simulink subsystem "Car"  (R2022b)
settings: Solver=VariableStepAuto  StartTime=0.0  StopTime=10.0  RelTol=1e-3
model mask{InitPos=0, InitVol=0}
  mask prompts: InitPos "Initial position (m)"; InitVol "Initial velocity (Km/hr)"
undefined symbols (not defined in the file or in its folder): DiscIntNeverNeededParam
settings Model: Creator=MAAM  LastModifiedBy=MAAM

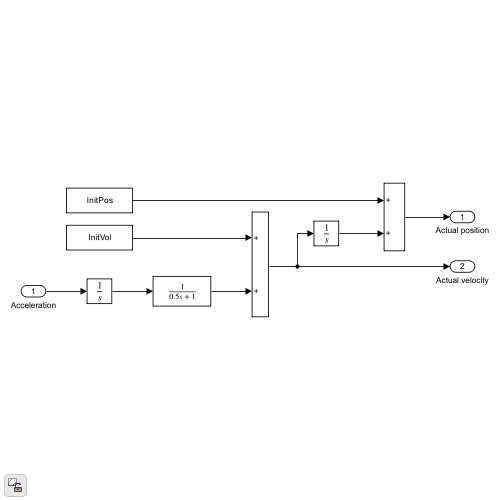
[thumbnail: Simulink's stored preview of the top-level diagram]
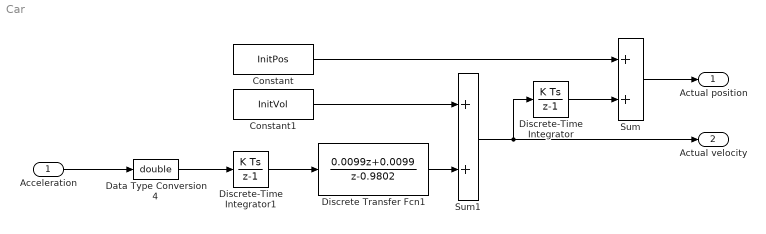
== system Car ==
  Acceleration : Inport
  Constant : Constant  Value=InitPos  OutDataTypeStr=Inherit: Inherit via back propagation  SampleTime=-1
  Constant1 : Constant  Value=InitVol  OutDataTypeStr=Inherit: Inherit via back propagation  SampleTime=-1
  Data Type Conversion4 : DataTypeConversion  OutDataTypeStr=double  SaturateOnIntegerOverflow=off  RndMeth=Floor
  Discrete Transfer Fcn1 : DiscreteTransferFcn  Numerator=[0.0099 0.0099]  Denominator=[1 -0.9802]  SampleTime=0.01
  Discrete-Time Integrator : DiscreteIntegrator  SampleTime=-1  ICPrevOutput=DiscIntNeverNeededParam  ICPrevScaledInput=DiscIntNeverNeededParam
  Discrete-Time Integrator1 : DiscreteIntegrator  SampleTime=-1  ICPrevOutput=DiscIntNeverNeededParam  ICPrevScaledInput=DiscIntNeverNeededParam
  Sum : Sum  OutDataTypeStr=Inherit: Inherit via back propagation
  Sum1 : Sum  OutDataTypeStr=Inherit: Inherit via back propagation
  Actual position : Outport  VectorParamsAs1DForOutWhenUnconnected=off
  Actual velocity : Outport  Port=2  VectorParamsAs1DForOutWhenUnconnected=off
  wires:
  Discrete-Time Integrator/1 -> Sum/2
  Constant/1 -> Sum/1
  Acceleration/1 -> Data Type Conversion4/1
  Sum1/1 -> Discrete-Time Integrator/1, Actual velocity/1
  Discrete-Time Integrator1/1 -> Discrete Transfer Fcn1/1
  Sum/1 -> Actual position/1
  Constant1/1 -> Sum1/1
  Discrete Transfer Fcn1/1 -> Sum1/2
  Data Type Conversion4/1 -> Discrete-Time Integrator1/1
